simulink model "SWC03_TrqCntrl"  (R2020b)
settings: Solver=FixedStepDiscrete  StartTime=0.0  StopTime=10.0  FixedStep=0.01  RelTol=1e-3
model workspace (MAT data in the model file):
  MSWC01_DrvLmt_Nm = Simulink.Parameter
  MSWC01_DrvLmt_Nm.Value = [225 225 225 225 205 190 175 165 150 140 130 122 116 112 108 106 104]
  MSWC01_DrvLmt_Nm.DataType = 'single'
  MSWC01_DrvLmt_Nm.DocUnits = 'N*m'
  MSWC01_DrvLmt_Nm.Dimensions = [1 17]
  MSWC01_FindBrk_Nm = Simulink.Parameter
  MSWC01_FindBrk_Nm.Value = [0 0 0 -20 -30 -40 -50 -60 -70 -80 -90 -95 -100 -100 -100 -100]
  MSWC01_FindBrk_Nm.DataType = 'single'
  MSWC01_FindBrk_Nm.DocUnits = 'N*m'
  MSWC01_FindBrk_Nm.Dimensions = [1 16]
  MSWC01_FindTrq_Nm = Simulink.Parameter
  MSWC01_FindTrq_Nm.Value = [0  0  0  0  -2  -4  -6  -8  -10  -14  -18  -22  -26  -30  -34  -38; 8  8  4  4  0  0  0  0  0  -10  -14  -18  -22  -26  -30  -34; 16  16  12  12  12  11  11  9  3  0  0  0  -18  -22  -26  -30; 48  48  46  46  45  42  36  25  17  13  11  5  0  0  0  -26; 73  71  69  67  63  60  54  42  30  25  22  19  15  12  11  0; 98  97  95  86  82  77  71  60  50  42  35  29  24  21  19  0; 119  117  115  105  105  100  95  89  79  69  59  48  39  29  27  0; 145  142  138  124  124  118  112  106  99  84  70  62  51  42  38  0; 174  167  154  150  150  146  140  132  122  108  95  78  63  55  47  0; 201  192  184  179  179  175  167  159  145  130  115  100  85  73  61  0; 225  225  223  223  223  220  220  198  172  153  138  120  104  99  86  0]
  MSWC01_FindTrq_Nm.DataType = 'single'
  MSWC01_FindTrq_Nm.DocUnits = 'N*m'
  MSWC01_FindTrq_Nm.Dimensions = [11 16]
  MSWC01_RegLmt_Nm = Simulink.Parameter
  MSWC01_RegLmt_Nm.Value = [-225 -225 -225 -225 -205 -190 -175 -165 -150 -140 -130 -122 -116 -112 -108 -106 -104]
  MSWC01_RegLmt_Nm.DataType = 'single'
  MSWC01_RegLmt_Nm.DocUnits = 'N*m'
  MSWC01_RegLmt_Nm.Dimensions = [1 17]
  NSWC05_ZeroTrq = 0
undefined symbols (not defined in the file): BrkOnPstn, BrkOnSpeed, C_0, C_1, C_100, C_m1, D, DRPMHigh, DRPMLow, DTempHigh, DTempLow, MCUMd_TC, R, SpeedDrtLmt
libraries: simulink x10
settings Model: OrderedModelArguments=off  Creator=Eric  LastModifiedBy=cyw40
settings OptimizationCC: BlockReduction=off  DefaultParameterBehavior=Inlined  UseDivisionForNetSlopeComputation=on  EnhancedBackFolding=on  PassReuseOutputArgsAs=Individual arguments  ZeroExternalMemoryAtStartup=off  ZeroInternalMemoryAtStartup=off  EfficientFloat2IntCast=on  OptimizeBlockOrder=speed  DifferentSizesBufferReuse=on  OptimizationCustomize=off  EfficientTunableParamExpr=on
settings DebuggingCC: SignalInfNanChecking=error  SignalRangeChecking=error  ReadBeforeWriteMsg=EnableAllAsError  WriteAfterWriteMsg=EnableAllAsError  WriteAfterReadMsg=EnableAllAsError  AlgebraicLoopMsg=error  ArtificialAlgebraicLoopMsg=error  SaveWithDisabledLinksMsg=error  SaveWithParameterizedLinksMsg=error  BlockPriorityViolationMsg=error  SolverPrmCheckMsg=error  InheritedTsInSrcMsg=error  SingleTaskRateTransMsg=error  TasksWithSamePriorityMsg=error  SigSpecEnsureSampleTimeMsg=error  CheckMatrixSingularityMsg=error  IntegerOverflowMsg=error  ParameterUnderflowMsg=error  ParameterPrecisionLossMsg=error  ParameterTunabilityLossMsg=error  UnderSpecifiedDataTypeMsg=error  UnnecessaryDatatypeConvMsg=warning  VectorMatrixConversionMsg=error  SignalLabelMismatchMsg=error  UnconnectedInputMsg=error  UnconnectedOutputMsg=error  UnconnectedLineMsg=error  SFcnCompatibilityMsg=error  UniqueDataStoreMsg=error  BusObjectLabelMismatch=error  RootOutportRequireBusObject=error  AssertControl=DisableAll  ModelReferenceIOMsg=error  ModelReferenceIOMismatchMessage=error  UnknownTsInhSupMsg=error  ModelReferenceDataLoggingMessage=error  StateNameClashWarn=warning  StrictBusMsg=ErrorOnBusTreatedAsVector  NonBusSignalsTreatedAsBus=error  SFInvalidInputDataAccessInChartInitDiag=error  SFTransitionOutsideNaturalParentDiag=error  SFUnreachableExecutionPathDiag=error  SFUndirectedBroadcastEventsDiag=error  SFTransitionActionBeforeConditionDiag=error  SFTemporalDelaySmallerThanSampleTimeDiag=error  SFSelfTransitionDiag=error  SFExecutionAtInitializationDiag=error  SFMachineParentedDataDiag=error  IntegerSaturationMsg=error
settings SFSimCC: CompileTimeRecursionLimit=0  EnableRuntimeRecursion=off  MATLABDynamicMemAlloc=off
settings RTWCC: Description=Embedded Coder  SystemTargetFile=ert.tlc  TemplateMakefile=ert_default_tmf
settings CodeAppCC: ForceParamTrailComments=on  IgnoreCustomStorageClasses=off  OperatorAnnotations=on  SimulinkDataObjDesc=on  SFDataObjDesc=on  MangleLength=4  InsertBlockDesc=on  ReqsInCode=on
settings ERTTargetCC: TargetLangStandard=C99 (ISO)  GenerateSampleERTMain=on  InlinedParameterPlacement=NonHierarchical  ERTCustomFileTemplate=example_file_process.tlc
settings ConfigComp: DVMode=DesignErrorDetection  DVTestSuiteOptimization=Auto  DVDetectActiveLogic=on  DVDetectInfNaN=on  DVDetectSubnormal=on  DVDesignMinMaxCheck=on  DVDetectHISMViolationsHisl_0002=on  DVDetectHISMViolationsHisl_0003=on  DVDetectHISMViolationsHisl_0004=on  DVDetectHISMViolationsHisl_0028=on  DVDetectBlockInputRangeViolations=on

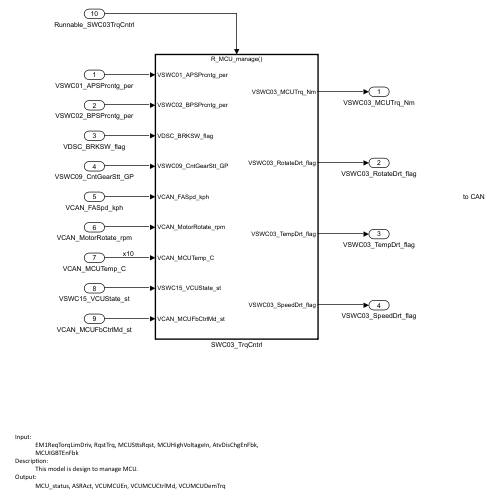
[thumbnail: Simulink's stored preview of the top-level diagram]
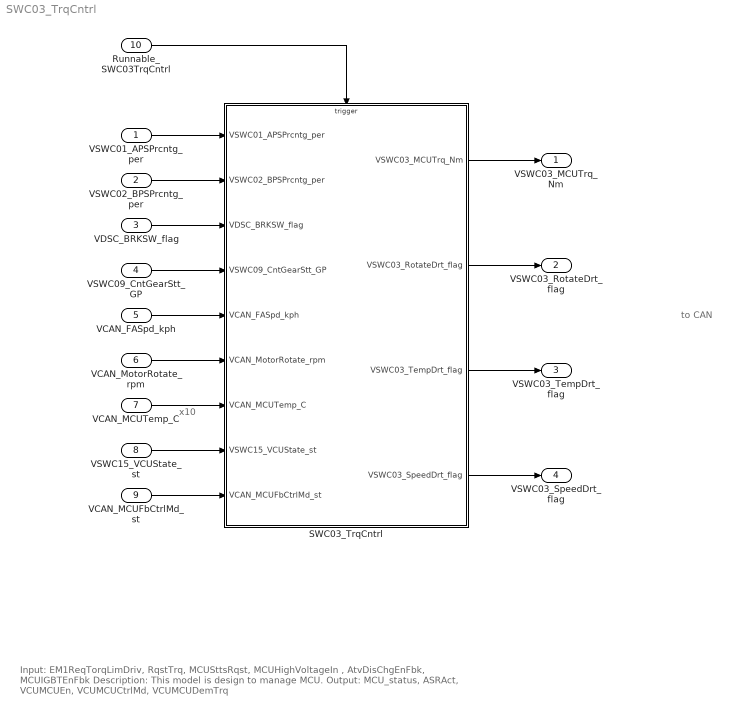
== system SWC03_TrqCntrl ==
  note: x10
  note: Input:
      | EM1ReqTorqLimDriv, RqstTrq, MCUSttsRqst, MCUHighVoltageIn , AtvDisChgEnFbk, MCUIGBTEnFbk
      | Description:
      | This model is design to manage MCU.
      | Output:
      | MCU_status, ASRAct, VCUMCUEn, VCUMCUCtrlMd, VCUMCUDemTrq
  note: to CAN
  VSWC01_APSPrcntg_per : Inport  OutMin=0  OutMax=100  OutDataTypeStr=uint8  Unit=%  PortDimensions=1
  VSWC02_BPSPrcntg_per : Inport  Port=2  OutMin=0  OutMax=100  OutDataTypeStr=uint8  Unit=%  PortDimensions=1
  VDSC_BRKSW_flag : Inport  Port=3  OutMin=0  OutMax=1  OutDataTypeStr=boolean  PortDimensions=1
  VSWC09_CntGearStt_GP : Inport  Port=4  OutMin=0  OutMax=4  OutDataTypeStr=uint8
  VCAN_FASpd_kph : Inport  Port=5  OutMin=0  OutMax=150  OutDataTypeStr=uint8  Unit=km/hr  PortDimensions=1
  VCAN_MotorRotate_rpm : Inport  Port=6  OutDataTypeStr=uint16
  VCAN_MCUTemp_C : Inport  Port=7  OutDataTypeStr=uint16
  VSWC15_VCUState_st : Inport  Port=8  OutDataTypeStr=uint8
  VCAN_MCUFbCtrlMd_st : Inport  Port=9  OutMin=0  OutMax=4  OutDataTypeStr=uint8  PortDimensions=1
  Runnable_SWC03TrqCntrl : Inport  Port=10  OutputFunctionCall=on
  SWC03_TrqCntrl : Subsystem
  VSWC03_MCUTrq_Nm : Outport
  VSWC03_RotateDrt_flag : Outport  Port=2
  VSWC03_TempDrt_flag : Outport  Port=3
  VSWC03_SpeedDrt_flag : Outport  Port=4
  wires:
  VSWC01_APSPrcntg_per/1 -> SWC03_TrqCntrl/1(VSWC01_APSPrcntg_per)
  Runnable_SWC03TrqCntrl/1 -> SWC03_TrqCntrl/Trigger
  VSWC02_BPSPrcntg_per/1 -> SWC03_TrqCntrl/2(VSWC02_BPSPrcntg_per)
  VSWC09_CntGearStt_GP/1 -> SWC03_TrqCntrl/4(VSWC09_CntGearStt_GP)
  VCAN_FASpd_kph/1 -> SWC03_TrqCntrl/5(VCAN_FASpd_kph)
  VCAN_MotorRotate_rpm/1 -> SWC03_TrqCntrl/6(VCAN_MotorRotate_rpm)
  VCAN_MCUTemp_C/1 -> SWC03_TrqCntrl/7(VCAN_MCUTemp_C)
  VSWC15_VCUState_st/1 -> SWC03_TrqCntrl/8(VSWC15_VCUState_st)
  VDSC_BRKSW_flag/1 -> SWC03_TrqCntrl/3(VDSC_BRKSW_flag)
  SWC03_TrqCntrl/1(VSWC03_MCUTrq_Nm) -> VSWC03_MCUTrq_Nm/1
  SWC03_TrqCntrl/2(VSWC03_RotateDrt_flag) -> VSWC03_RotateDrt_flag/1
  SWC03_TrqCntrl/4(VSWC03_SpeedDrt_flag) -> VSWC03_SpeedDrt_flag/1
  SWC03_TrqCntrl/3(VSWC03_TempDrt_flag) -> VSWC03_TempDrt_flag/1
  VCAN_MCUFbCtrlMd_st/1 -> SWC03_TrqCntrl/9(VCAN_MCUFbCtrlMd_st)

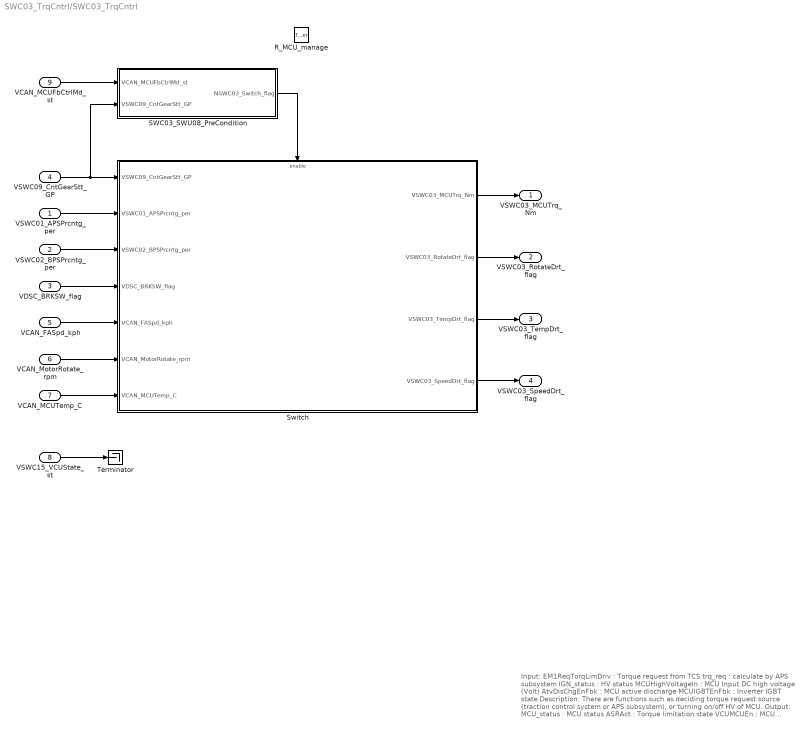
== system SWC03_TrqCntrl/SWC03_TrqCntrl ==
  note: Input:
      | EM1ReqTorqLimDriv : Torque request from TCS
      | trq_req : calculate by APS subsystem
      | IGN_status : HV status
      | MCUHighVoltageIn : MCU Input DC high voltage (Volt)
      | AtvDisChgEnFbk : MCU active discharge
      | MCUIGBTEnFbk : Inverter IGBT state
      | Description:
      | There are functions such as
      | deciding torque request source (traction control system or APS subsystem),
      | or turning on/off HV of MCU.
      | Output:
      | MCU_status : MCU status
      | ASRAct : Torque limitation state
      | VCUMCUEn : MCU enable command
      | VCUMCUCtrlMd : Operation mode of MCU
      | VCUMCUDemTrq : Torque request of traction motor (Nm)
  VSWC01_APSPrcntg_per : Inport
  VSWC02_BPSPrcntg_per : Inport  Port=2
  VDSC_BRKSW_flag : Inport  Port=3
  VSWC09_CntGearStt_GP : Inport  Port=4
  VCAN_FASpd_kph : Inport  Port=5
  VCAN_MotorRotate_rpm : Inport  Port=6
  VCAN_MCUTemp_C : Inport  Port=7
  VSWC15_VCUState_st : Inport  Port=8
  VCAN_MCUFbCtrlMd_st : Inport  Port=9
  R_MCU_manage : TriggerPort  TriggerType=function-call  VariantControl=(inherit)
  SWC03_SWU08_PreCondition : Subsystem  TreatAsAtomicUnit=on  RTWFcnName=SWC03_SWU08_PreCondition
      settings: RTWFcnNameOpts=User specified
  Switch : Subsystem
  Terminator : Terminator
  VSWC03_MCUTrq_Nm : Outport
  VSWC03_RotateDrt_flag : Outport  Port=2
  VSWC03_TempDrt_flag : Outport  Port=3
  VSWC03_SpeedDrt_flag : Outport  Port=4
  wires:
  VSWC01_APSPrcntg_per/1 -> Switch/2(VSWC01_APSPrcntg_per)
  VSWC02_BPSPrcntg_per/1 -> Switch/3(VSWC02_BPSPrcntg_per)
  VSWC09_CntGearStt_GP/1 -> SWC03_SWU08_PreCondition/2(VSWC09_CntGearStt_GP), Switch/1(VSWC09_CntGearStt_GP)
  VCAN_FASpd_kph/1 -> Switch/5(VCAN_FASpd_kph)
  VDSC_BRKSW_flag/1 -> Switch/4(VDSC_BRKSW_flag)
  VCAN_MotorRotate_rpm/1 -> Switch/6(VCAN_MotorRotate_rpm)
  VCAN_MCUTemp_C/1 -> Switch/7(VCAN_MCUTemp_C)
  Switch/1(VSWC03_MCUTrq_Nm) -> VSWC03_MCUTrq_Nm/1
  Switch/2(VSWC03_RotateDrt_flag) -> VSWC03_RotateDrt_flag/1
  Switch/4(VSWC03_SpeedDrt_flag) -> VSWC03_SpeedDrt_flag/1
  Switch/3(VSWC03_TempDrt_flag) -> VSWC03_TempDrt_flag/1
  VCAN_MCUFbCtrlMd_st/1 -> SWC03_SWU08_PreCondition/1(VCAN_MCUFbCtrlMd_st)
  SWC03_SWU08_PreCondition/1(NSWC03_Switch_flag) -> Switch/Enable
  VSWC15_VCUState_st/1 -> Terminator/1

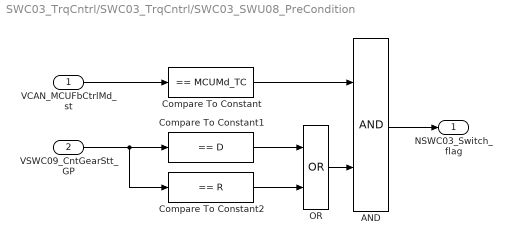
== system SWC03_TrqCntrl/SWC03_TrqCntrl/SWC03_SWU08_PreCondition ==
  VCAN_MCUFbCtrlMd_st : Inport
  VSWC09_CntGearStt_GP : Inport  Port=2
  AND : Logic  AllPortsSameDT=off  OutDataTypeStr=boolean
  Compare To Constant : simulink/Logic and Bit Operations/Compare To Constant  relop===  const=MCUMd_TC  OutDataTypeStr=boolean
  Compare To Constant1 : simulink/Logic and Bit Operations/Compare To Constant  relop===  const=D  OutDataTypeStr=boolean
  Compare To Constant2 : simulink/Logic and Bit Operations/Compare To Constant  relop===  const=R  OutDataTypeStr=boolean
  OR : Logic  Operator=OR  AllPortsSameDT=off  OutDataTypeStr=boolean
  NSWC03_Switch_flag : Outport
  wires:
  VSWC09_CntGearStt_GP/1 -> Compare To Constant2/1, Compare To Constant1/1
  Compare To Constant1/1 -> OR/1
  Compare To Constant2/1 -> OR/2
  VCAN_MCUFbCtrlMd_st/1 -> Compare To Constant/1
  OR/1 -> AND/2
  Compare To Constant/1 -> AND/1
  AND/1 -> NSWC03_Switch_flag/1

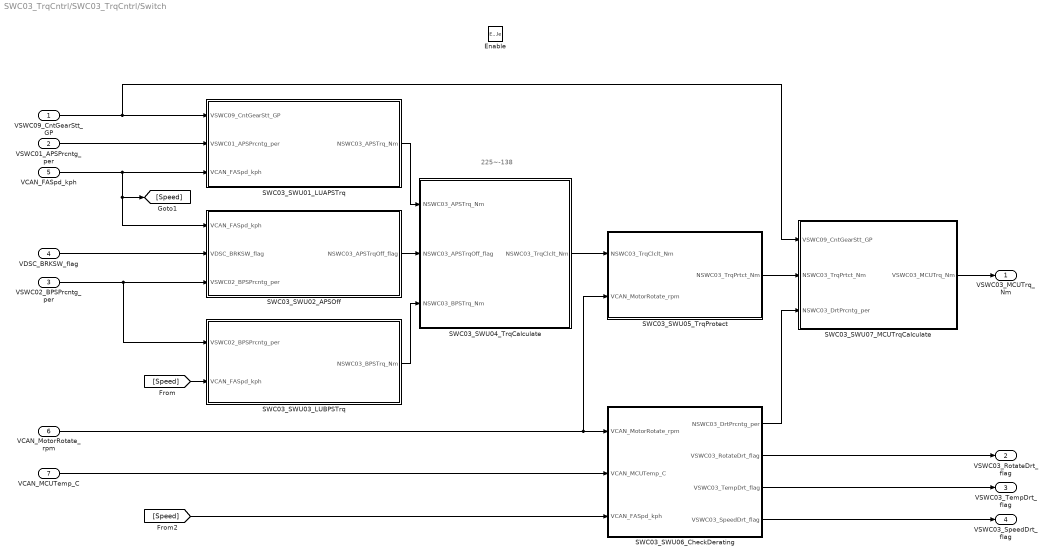
== system SWC03_TrqCntrl/SWC03_TrqCntrl/Switch ==
  note: 225~-138
  VSWC09_CntGearStt_GP : Inport
  VSWC01_APSPrcntg_per : Inport  Port=2
  VSWC02_BPSPrcntg_per : Inport  Port=3
  VDSC_BRKSW_flag : Inport  Port=4
  VCAN_FASpd_kph : Inport  Port=5
  VCAN_MotorRotate_rpm : Inport  Port=6
  VCAN_MCUTemp_C : Inport  Port=7
  Enable : EnablePort  StatesWhenEnabling=reset
  SWC03_SWU01_LUAPSTrq : Subsystem  TreatAsAtomicUnit=on  RTWFcnName=SWC03_SWU01_LUAPSTrq
      settings: RTWFcnNameOpts=User specified
  SWC03_SWU02_APSOff : Subsystem  TreatAsAtomicUnit=on  RTWFcnName=SWC03_SWU02_APSOff
      settings: RTWFcnNameOpts=User specified
  SWC03_SWU03_LUBPSTrq : Subsystem  TreatAsAtomicUnit=on  RTWFcnName=SWC03_SWU03_LUBPSTrq
      settings: RTWFcnNameOpts=User specified
  SWC03_SWU04_TrqCalculate : Subsystem  TreatAsAtomicUnit=on  RTWFcnName=SWC03_SWU04_TrqCalculate
      settings: RTWFcnNameOpts=User specified
  SWC03_SWU05_TrqProtect : Subsystem  TreatAsAtomicUnit=on  RTWFcnName=SWC03_SWU06_TrqProtect
      settings: RTWFcnNameOpts=User specified
  SWC03_SWU06_CheckDerating : Subsystem  TreatAsAtomicUnit=on  RTWFcnName=SWC03_SWU05_CheckDerating
      settings: RTWFcnNameOpts=User specified
  SWC03_SWU07_MCUTrqCalculate : Subsystem  TreatAsAtomicUnit=on  RTWFcnName=SWC03_SWU07_MCUTrqCalculate
      settings: RTWFcnNameOpts=User specified
  VSWC03_MCUTrq_Nm : Outport  OutputWhenDisabled=reset  InitialOutput=0
  VSWC03_RotateDrt_flag : Outport  Port=2  OutputWhenDisabled=reset  InitialOutput=false
  VSWC03_TempDrt_flag : Outport  Port=3  OutputWhenDisabled=reset  InitialOutput=false
  VSWC03_SpeedDrt_flag : Outport  Port=4  OutputWhenDisabled=reset  InitialOutput=false
  wires:
  VCAN_FASpd_kph/1 -> SWC03_SWU02_APSOff/1(VCAN_FASpd_kph), [Speed], SWC03_SWU01_LUAPSTrq/3(VCAN_FASpd_kph)
  VSWC01_APSPrcntg_per/1 -> SWC03_SWU01_LUAPSTrq/2(VSWC01_APSPrcntg_per)
  VSWC02_BPSPrcntg_per/1 -> SWC03_SWU02_APSOff/3(VSWC02_BPSPrcntg_per), SWC03_SWU03_LUBPSTrq/1(VSWC02_BPSPrcntg_per)
  VDSC_BRKSW_flag/1 -> SWC03_SWU02_APSOff/2(VDSC_BRKSW_flag)
  [Speed] -> SWC03_SWU03_LUBPSTrq/2(VCAN_FASpd_kph)
  SWC03_SWU01_LUAPSTrq/1(NSWC03_APSTrq_Nm) -> SWC03_SWU04_TrqCalculate/1(NSWC03_APSTrq_Nm)
  SWC03_SWU02_APSOff/1(NSWC03_APSTrqOff_flag) -> SWC03_SWU04_TrqCalculate/2(NSWC03_APSTrqOff_flag)
  SWC03_SWU03_LUBPSTrq/1(NSWC03_BPSTrq_Nm) -> SWC03_SWU04_TrqCalculate/3(NSWC03_BPSTrq_Nm)
  VCAN_MotorRotate_rpm/1 -> SWC03_SWU06_CheckDerating/1(VCAN_MotorRotate_rpm), SWC03_SWU05_TrqProtect/2(VCAN_MotorRotate_rpm)
  SWC03_SWU04_TrqCalculate/1(NSWC03_TrqClclt_Nm) -> SWC03_SWU05_TrqProtect/1(NSWC03_TrqClclt_Nm)
  VCAN_MCUTemp_C/1 -> SWC03_SWU06_CheckDerating/2(VCAN_MCUTemp_C)
  [Speed] -> SWC03_SWU06_CheckDerating/3(VCAN_FASpd_kph)
  SWC03_SWU06_CheckDerating/4(VSWC03_SpeedDrt_flag) -> VSWC03_SpeedDrt_flag/1
  SWC03_SWU06_CheckDerating/3(VSWC03_TempDrt_flag) -> VSWC03_TempDrt_flag/1
  SWC03_SWU05_TrqProtect/1(NSWC03_TrqPrtct_Nm) -> SWC03_SWU07_MCUTrqCalculate/2(NSWC03_TrqPrtct_Nm)
  VSWC09_CntGearStt_GP/1 -> SWC03_SWU07_MCUTrqCalculate/1(VSWC09_CntGearStt_GP), SWC03_SWU01_LUAPSTrq/1(VSWC09_CntGearStt_GP)
  SWC03_SWU06_CheckDerating/2(VSWC03_RotateDrt_flag) -> VSWC03_RotateDrt_flag/1
  SWC03_SWU06_CheckDerating/1(NSWC03_DrtPrcntg_per) -> SWC03_SWU07_MCUTrqCalculate/3(NSWC03_DrtPrcntg_per)
  SWC03_SWU07_MCUTrqCalculate/1(VSWC03_MCUTrq_Nm) -> VSWC03_MCUTrq_Nm/1

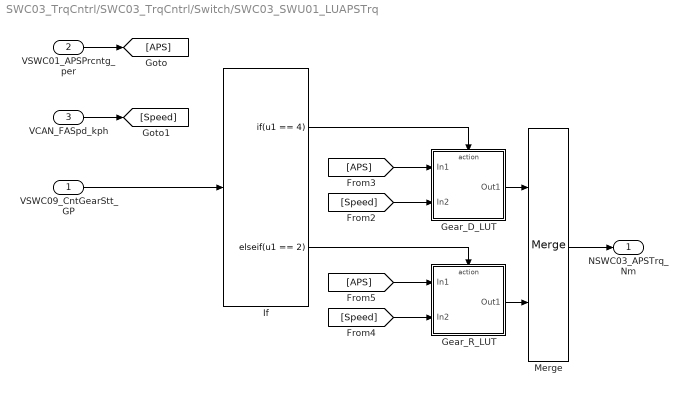
== system SWC03_TrqCntrl/SWC03_TrqCntrl/Switch/SWC03_SWU01_LUAPSTrq ==
  VSWC09_CntGearStt_GP : Inport
  VSWC01_APSPrcntg_per : Inport  Port=2
  VCAN_FASpd_kph : Inport  Port=3
  Gear_D_LUT : Subsystem  TreatAsAtomicUnit=on
      mask Display: image('D.png'); % Use "Edit Image" on toolstrip to change.
  Gear_R_LUT : Subsystem  TreatAsAtomicUnit=on
      mask Display: image('R.png'); % Use "Edit Image" on toolstrip to change.
  If : If  IfExpression=u1 == 4  ElseIfExpressions=u1 == 2  ShowElse=off
  Merge : Merge
  NSWC03_APSTrq_Nm : Outport
  wires:
  Gear_R_LUT/1(Out1) -> Merge/2
  [APS] -> Gear_R_LUT/1(In1)
  [Speed] -> Gear_D_LUT/2(In2)
  If/1 -> Gear_D_LUT/Action
  [APS] -> Gear_D_LUT/1(In1)
  [Speed] -> Gear_R_LUT/2(In2)
  VSWC09_CntGearStt_GP/1 -> If/1
  If/2 -> Gear_R_LUT/Action
  Gear_D_LUT/1(Out1) -> Merge/1
  Merge/1 -> NSWC03_APSTrq_Nm/1
  VSWC01_APSPrcntg_per/1 -> [APS]
  VCAN_FASpd_kph/1 -> [Speed]

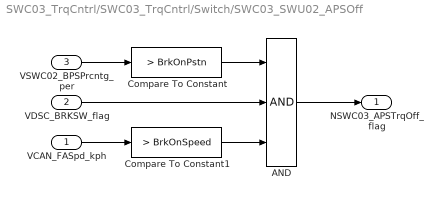
== system SWC03_TrqCntrl/SWC03_TrqCntrl/Switch/SWC03_SWU02_APSOff ==
  VCAN_FASpd_kph : Inport
  VDSC_BRKSW_flag : Inport  Port=2
  VSWC02_BPSPrcntg_per : Inport  Port=3
  AND : Logic  Inputs=3  AllPortsSameDT=off  OutDataTypeStr=boolean
  Compare To Constant : simulink/Logic and Bit Operations/Compare To Constant  relop=>  const=BrkOnPstn  OutDataTypeStr=boolean
  Compare To Constant1 : simulink/Logic and Bit Operations/Compare To Constant  relop=>  const=BrkOnSpeed  OutDataTypeStr=boolean
  NSWC03_APSTrqOff_flag : Outport
  wires:
  AND/1 -> NSWC03_APSTrqOff_flag/1
  VSWC02_BPSPrcntg_per/1 -> Compare To Constant/1
  VCAN_FASpd_kph/1 -> Compare To Constant1/1
  VDSC_BRKSW_flag/1 -> AND/2
  Compare To Constant/1 -> AND/1
  Compare To Constant1/1 -> AND/3

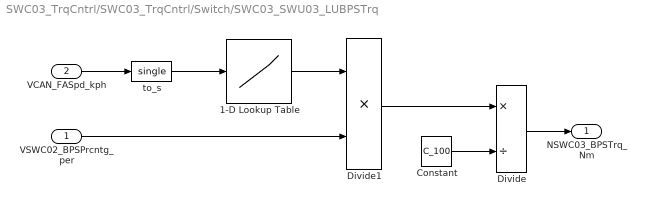
== system SWC03_TrqCntrl/SWC03_TrqCntrl/Switch/SWC03_SWU03_LUBPSTrq ==
  VSWC02_BPSPrcntg_per : Inport
  VCAN_FASpd_kph : Inport  Port=2
  1-D Lookup Table : Lookup_n-D  NumberOfTableDimensions=1  BreakpointsForDimension1=[0:10:150]  BreakpointsForDimension1DataTypeStr=single  Table=MSWC01_FindBrk_Nm  TableDataTypeStr=single  IntermediateResultsDataTypeStr=single  InternalRulePriority=Speed  OutDataTypeStr=single  RndMeth=Simplest  FractionDataTypeStr=single  InputSameDT=on
  Constant : Constant  Value=C_100  OutDataTypeStr=single  SampleTime=-1
  Divide : Product  Inputs=*/
  Divide1 : Product  Inputs=**
  to_s : DataTypeConversion  OutDataTypeStr=single
  NSWC03_BPSTrq_Nm : Outport
  wires:
  VCAN_FASpd_kph/1 -> to_s/1
  to_s/1 -> 1-D Lookup Table/1
  VSWC02_BPSPrcntg_per/1 -> Divide1/2
  1-D Lookup Table/1 -> Divide1/1
  Divide1/1 -> Divide/1
  Constant/1 -> Divide/2
  Divide/1 -> NSWC03_BPSTrq_Nm/1

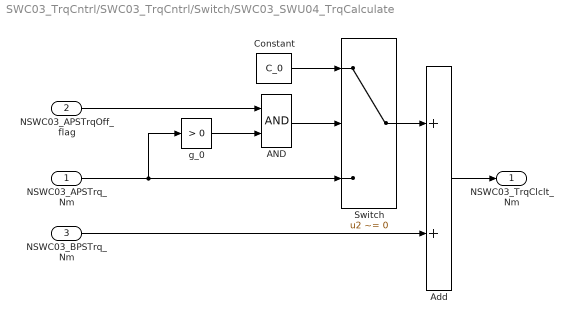
== system SWC03_TrqCntrl/SWC03_TrqCntrl/Switch/SWC03_SWU04_TrqCalculate ==
  NSWC03_APSTrq_Nm : Inport
  NSWC03_APSTrqOff_flag : Inport  Port=2
  NSWC03_BPSTrq_Nm : Inport  Port=3
  AND : Logic  AllPortsSameDT=off  OutDataTypeStr=boolean
  Add : Sum
  Constant : Constant  Value=C_0  OutDataTypeStr=single  SampleTime=-1
  Switch : Switch  Criteria=u2 ~= 0
  g_0 : simulink/Logic and Bit Operations/Compare To Constant  relop=>  const=0  OutDataTypeStr=boolean
  NSWC03_TrqClclt_Nm : Outport
  wires:
  Add/1 -> NSWC03_TrqClclt_Nm/1
  Switch/1 -> Add/1
  NSWC03_BPSTrq_Nm/1 -> Add/2
  Constant/1 -> Switch/1
  NSWC03_APSTrq_Nm/1 -> g_0/1, Switch/3
  AND/1 -> Switch/2
  g_0/1 -> AND/2
  NSWC03_APSTrqOff_flag/1 -> AND/1

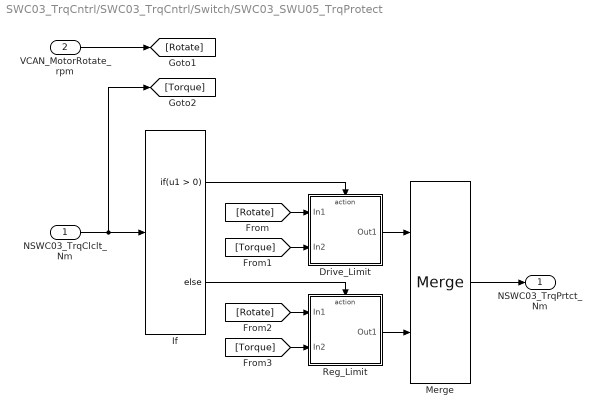
== system SWC03_TrqCntrl/SWC03_TrqCntrl/Switch/SWC03_SWU05_TrqProtect ==
  NSWC03_TrqClclt_Nm : Inport
  VCAN_MotorRotate_rpm : Inport  Port=2
  Drive_Limit : Subsystem  TreatAsAtomicUnit=on
  If : If
  Merge : Merge
  Reg_Limit : Subsystem  TreatAsAtomicUnit=on
  NSWC03_TrqPrtct_Nm : Outport
  wires:
  If/1 -> Drive_Limit/Action
  NSWC03_TrqClclt_Nm/1 -> [Torque], If/1
  VCAN_MotorRotate_rpm/1 -> [Rotate]
  If/2 -> Reg_Limit/Action
  [Rotate] -> Drive_Limit/1(In1)
  [Torque] -> Drive_Limit/2(In2)
  [Rotate] -> Reg_Limit/1(In1)
  [Torque] -> Reg_Limit/2(In2)
  Drive_Limit/1(Out1) -> Merge/1
  Reg_Limit/1(Out1) -> Merge/2
  Merge/1 -> NSWC03_TrqPrtct_Nm/1

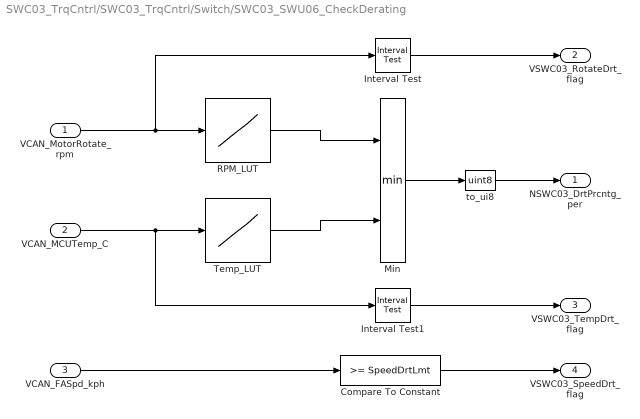
== system SWC03_TrqCntrl/SWC03_TrqCntrl/Switch/SWC03_SWU06_CheckDerating ==
  VCAN_MotorRotate_rpm : Inport
  VCAN_MCUTemp_C : Inport  Port=2
  VCAN_FASpd_kph : Inport  Port=3
  Compare To Constant : simulink/Logic and Bit Operations/Compare To Constant  relop=>=  const=SpeedDrtLmt  OutDataTypeStr=boolean
  Interval Test : simulink/Logic and Bit Operations/Interval Test  IntervalClosedRight=on  uplimit=DRPMHigh  IntervalClosedLeft=on  lowlimit=DRPMLow  OutDataTypeStr=boolean
      settings: AttributesFormatString=%<uplimit>~%<lowlimit>
  Interval Test1 : simulink/Logic and Bit Operations/Interval Test  IntervalClosedRight=on  uplimit=DTempHigh  IntervalClosedLeft=on  lowlimit=DTempLow  OutDataTypeStr=boolean
      settings: AttributesFormatString=%<uplimit>~%<lowlimit>
  Min : MinMax  Inputs=2
  RPM_LUT : Lookup_n-D  NumberOfTableDimensions=1  BreakpointsForDimension1=[15000:10:16000]  BreakpointsForDimension1DataTypeStr=uint16  Table=100 - [0:100]  TableDataTypeStr=uint16  IntermediateResultsDataTypeStr=single  InterpMethod=Flat  ExtrapMethod=Clip  UseLastTableValue=on  InternalRulePriority=Speed  OutDataTypeStr=uint16  RndMeth=Simplest  FractionDataTypeStr=single  InputSameDT=on
  Temp_LUT : Lookup_n-D  NumberOfTableDimensions=1  BreakpointsForDimension1=[1250:1350]  BreakpointsForDimension1DataTypeStr=uint16  Table=100 - [0:100]  TableDataTypeStr=uint16  IntermediateResultsDataTypeStr=single  InterpMethod=Flat  ExtrapMethod=Clip  UseLastTableValue=on  InternalRulePriority=Speed  OutDataTypeStr=uint16  RndMeth=Simplest  FractionDataTypeStr=single  InputSameDT=on
  to_ui8 : DataTypeConversion  OutDataTypeStr=uint8
  NSWC03_DrtPrcntg_per : Outport
  VSWC03_RotateDrt_flag : Outport  Port=2
  VSWC03_TempDrt_flag : Outport  Port=3
  VSWC03_SpeedDrt_flag : Outport  Port=4
  wires:
  to_ui8/1 -> NSWC03_DrtPrcntg_per/1
  VCAN_MotorRotate_rpm/1 -> Interval Test/1, RPM_LUT/1
  VCAN_MCUTemp_C/1 -> Temp_LUT/1, Interval Test1/1
  VCAN_FASpd_kph/1 -> Compare To Constant/1
  Compare To Constant/1 -> VSWC03_SpeedDrt_flag/1
  Interval Test/1 -> VSWC03_RotateDrt_flag/1
  Interval Test1/1 -> VSWC03_TempDrt_flag/1
  RPM_LUT/1 -> Min/1
  Temp_LUT/1 -> Min/2
  Min/1 -> to_ui8/1

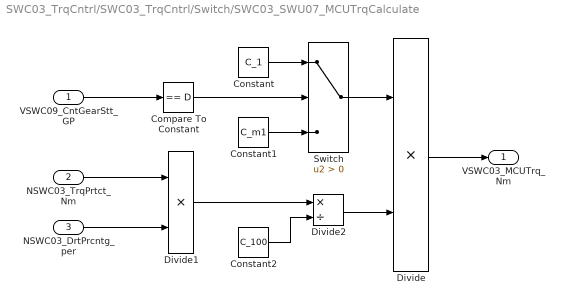
== system SWC03_TrqCntrl/SWC03_TrqCntrl/Switch/SWC03_SWU07_MCUTrqCalculate ==
  VSWC09_CntGearStt_GP : Inport
  NSWC03_TrqPrtct_Nm : Inport  Port=2
  NSWC03_DrtPrcntg_per : Inport  Port=3
  Compare To Constant : simulink/Logic and Bit Operations/Compare To Constant  relop===  const=D  OutDataTypeStr=boolean
  Constant : Constant  Value=C_1  OutDataTypeStr=int8  SampleTime=-1
  Constant1 : Constant  Value=C_m1  OutDataTypeStr=int8  SampleTime=-1
  Constant2 : Constant  Value=C_100  OutDataTypeStr=uint8
  Divide : Product  Inputs=**
  Divide1 : Product  Inputs=**
  Divide2 : Product  Inputs=*/
  Switch : Switch  Criteria=u2 > Threshold
  VSWC03_MCUTrq_Nm : Outport
  wires:
  Switch/1 -> Divide/1
  VSWC09_CntGearStt_GP/1 -> Compare To Constant/1
  Constant/1 -> Switch/1
  Constant1/1 -> Switch/3
  NSWC03_DrtPrcntg_per/1 -> Divide1/2
  NSWC03_TrqPrtct_Nm/1 -> Divide1/1
  Compare To Constant/1 -> Switch/2
  Divide1/1 -> Divide2/1
  Constant2/1 -> Divide2/2
  Divide2/1 -> Divide/2
  Divide/1 -> VSWC03_MCUTrq_Nm/1

== system SWC03_TrqCntrl/SWC03_TrqCntrl/Switch/SWC03_SWU01_LUAPSTrq/Gear_D_LUT ==
  In1 : Inport
  In2 : Inport  Port=2
  Action Port : ActionPort  ActionPortLabel=if(u1 == 4)
  APS_Spd_D : Lookup_n-D  BreakpointsForDimension1=[0:10:100]  BreakpointsForDimension2=[0:10:150]  BreakpointsForDimension1DataTypeStr=single  BreakpointsForDimension2DataTypeStr=single  Table=MSWC01_FindTrq_Nm  TableDataTypeStr=single  IntermediateResultsDataTypeStr=single  ExtrapMethod=Clip  UseLastTableValue=on  InternalRulePriority=Speed  OutDataTypeStr=single  InputSameDT=on
      settings: AttributesFormatString=UseLastTableValue=%<UseLastTableValue>  InputPortMap=u0,u1
  Out1 : Outport
  wires:
  In1/1 -> APS_Spd_D/1
  In2/1 -> APS_Spd_D/2
  APS_Spd_D/1 -> Out1/1

== system SWC03_TrqCntrl/SWC03_TrqCntrl/Switch/SWC03_SWU01_LUAPSTrq/Gear_R_LUT ==
  In1 : Inport
  In2 : Inport  Port=2
  Action Port : ActionPort  ActionPortLabel=elseif(u1 == 2)
  APS_Spd_R : Lookup_n-D  BreakpointsForDimension1=[0:10:100]  BreakpointsForDimension2=[0:10:150]  BreakpointsForDimension1DataTypeStr=single  BreakpointsForDimension2DataTypeStr=single  Table=MSWC01_FindTrq_Nm  TableDataTypeStr=single  IntermediateResultsDataTypeStr=single  ExtrapMethod=Clip  UseLastTableValue=on  InternalRulePriority=Speed  OutDataTypeStr=single  InputSameDT=on
      settings: AttributesFormatString=UseLastTableValue=%<UseLastTableValue>  InputPortMap=u0,u1
  Out1 : Outport
  wires:
  In1/1 -> APS_Spd_R/1
  In2/1 -> APS_Spd_R/2
  APS_Spd_R/1 -> Out1/1

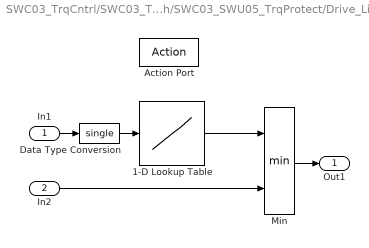
== system SWC03_TrqCntrl/SWC03_TrqCntrl/Switch/SWC03_SWU05_TrqProtect/Drive_Limit ==
  In1 : Inport
  In2 : Inport  Port=2
  Action Port : ActionPort  ActionPortLabel=if(u1 > 0)
  1-D Lookup Table : Lookup_n-D  NumberOfTableDimensions=1  BreakpointsForDimension1=[0:1000:16000]  BreakpointsForDimension1DataTypeStr=single  Table=MSWC01_DrvLmt_Nm  TableDataTypeStr=single  IntermediateResultsDataTypeStr=single  InternalRulePriority=Speed  OutDataTypeStr=single  RndMeth=Simplest  FractionDataTypeStr=single  InputSameDT=on
  Data Type Conversion : DataTypeConversion  OutDataTypeStr=single
  Min : MinMax  Inputs=2
  Out1 : Outport
  wires:
  In1/1 -> Data Type Conversion/1
  1-D Lookup Table/1 -> Min/1
  In2/1 -> Min/2
  Min/1 -> Out1/1
  Data Type Conversion/1 -> 1-D Lookup Table/1

== system SWC03_TrqCntrl/SWC03_TrqCntrl/Switch/SWC03_SWU05_TrqProtect/Reg_Limit ==
  In1 : Inport
  In2 : Inport  Port=2
  Action Port : ActionPort  ActionPortLabel=else
  1-D Lookup Table : Lookup_n-D  NumberOfTableDimensions=1  BreakpointsForDimension1=[0:1000:16000]  BreakpointsForDimension1DataTypeStr=single  Table=MSWC01_RegLmt_Nm  TableDataTypeStr=single  IntermediateResultsDataTypeStr=single  InternalRulePriority=Speed  OutDataTypeStr=single  RndMeth=Simplest  FractionDataTypeStr=single  InputSameDT=on
  Data Type Conversion : DataTypeConversion  OutDataTypeStr=single
  Max : MinMax  Function=max  Inputs=2
  Out1 : Outport
  wires:
  In1/1 -> Data Type Conversion/1
  1-D Lookup Table/1 -> Max/1
  In2/1 -> Max/2
  Max/1 -> Out1/1
  Data Type Conversion/1 -> 1-D Lookup Table/1
